simulink model "LIF_Na"  (R2025a)
settings: Solver=ode45  StartTime=0.0  StopTime=0.5  MaxStep=0.00001  RelTol=1e-3
undefined symbols (not defined in the file): ahp_strength, C_m, E_L, g_ahp, R_m, tau_ahp, V_reset, V_th
settings Model: Creator=pradipkumarde  LastModifiedBy=pradipkumarde

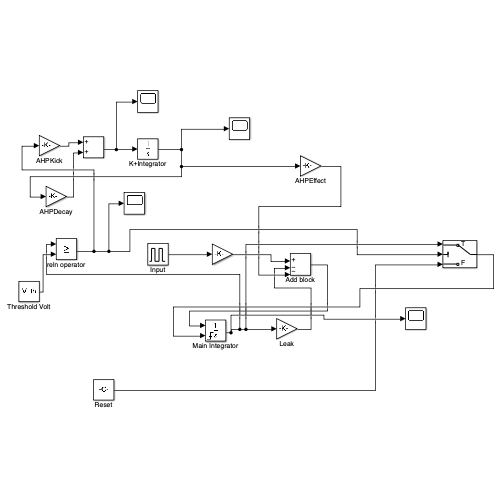
[thumbnail: Simulink's stored preview of the top-level diagram]
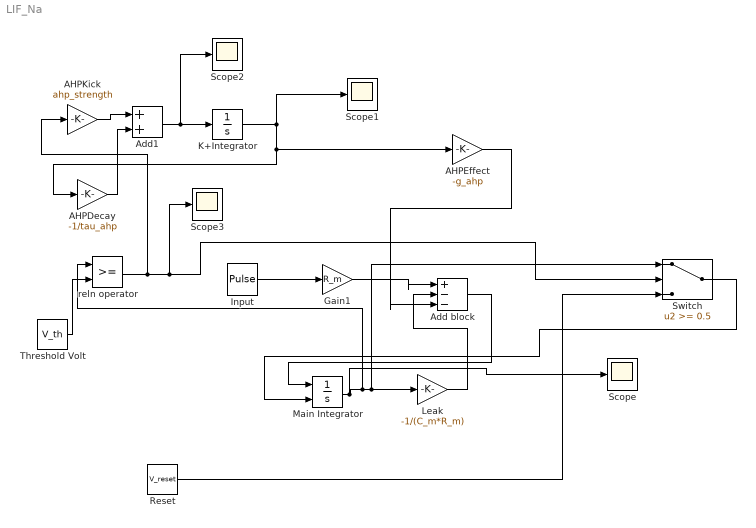
== system LIF_Na ==
  AHPDecay : Gain  Gain=-1/tau_ahp
  AHPEffect : Gain  Gain=-g_ahp
  AHPKick : Gain  Gain=ahp_strength
  Add block : Sum  Inputs=|+--
  Add1 : Sum
  Gain1 : Gain  Gain=R_m
  Input : DiscretePulseGenerator  PulseType=Time based  Amplitude=10e-9  Period=0.1  PulseWidth=50
  K+Integrator : Integrator
  Leak : Gain  Gain=-1/(C_m*R_m)
  Main Integrator : Integrator  ExternalReset=rising  InitialCondition=E_L
  Reset : Constant  Value=V_reset
  Scope{,1..3} (4 alike) : Scope
      Scope settings: ActiveDisplayYMinimum=-0.10249204401131068  ActiveDisplayYMaximum=0.10585628213400555
      Scope1 settings: ActiveDisplayYMinimum=-1  ActiveDisplayYMaximum=1
      Scope2 settings: ActiveDisplayYMinimum=-1  ActiveDisplayYMaximum=1  DataLoggingVariableName=ScopeData2
      Scope3 settings: ActiveDisplayYMinimum=-1  ActiveDisplayYMaximum=1  DataLoggingVariableName=ScopeData3
  Switch : Switch  Threshold=0.5  SaturateOnIntegerOverflow=off  InputSameDT=off
  Threshold Volt : Constant  Value=V_th
  reln operator : RelationalOperator  OutDataTypeStr=boolean  RndMeth=Simplest  InputSameDT=off
  wires:
  Input/1 -> Gain1/1
  Gain1/1 -> Add block/1
  Main Integrator/1 -> Scope/1, reln operator/1, Switch/1, Leak/1
  Leak/1 -> Add block/2
  Add block/1 -> Main Integrator/1
  Threshold Volt/1 -> reln operator/2
  Reset/1 -> Switch/3
  reln operator/1 -> AHPKick/1, Scope3/1, Switch/2
  Switch/1 -> Main Integrator/2
  AHPKick/1 -> Add1/1
  AHPDecay/1 -> Add1/2
  Add1/1 -> Scope2/1, K+Integrator/1
  K+Integrator/1 -> AHPEffect/1, AHPDecay/1, Scope1/1
  AHPEffect/1 -> Add block/3
